simulink model "momentumBasedFlight"  (R2021b)
settings: Solver=FixedStepDiscrete  StartTime=0.0  StopTime=Config.simulationTime  FixedStep=Config.tStep  RelTol=1e-3
InitFcn:
  | cd(fileparts(which(bdroot)));
  | initMomentumBasedFlight;
StopFcn:
  | cd(fileparts(which(bdroot)));
  | stopMomentumBasedFlight;
undefined symbols (not defined in the file or in its folder): Config
libraries: WBToolboxLibrary x18, momentum_flight_control_v1 x6, thrust_estimation_v1 x1, jets_control_v1 x1
settings Model: NumberOfSteps=50  Creator=gnava  LastModifiedBy=gnava
settings SolverCC: AlgebraicLoopSolver=TrustRegion
settings DataIOCC: ReturnWorkspaceOutputs=off
settings OptimizationCC: BlockReduction=off  DefaultParameterBehavior=Inlined  BufferReuse=off
settings DebuggingCC: SFMachineParentedDataDiag=warning  ArithmeticOperatorsInVariantConditions=warning
settings SFSimCC: SimUseLocalCustomCode=off  CustomCodeUndefinedFunction=UseInterfaceOnly
settings RTWCC: RTWUseLocalCustomCode=off

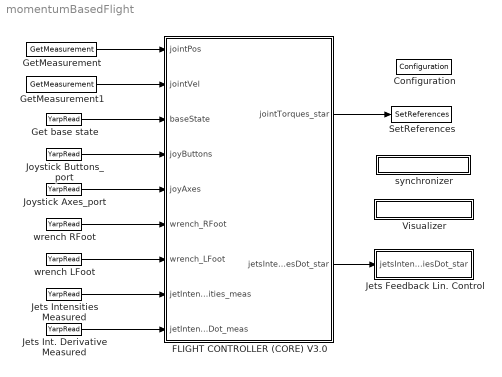
== system momentumBasedFlight ==
  Configuration : WBToolboxLibrary/Utilities/Configuration  ConfigSource=Workspace  ConfigObject='WBTConfigRobot'  RobotName='icubSim'  UrdfFile='model.urdf'  ControlledJoints={'l_elbow','l_shoulder_pitch','torso_roll'}  ControlBoardsNames={'left_arm','right_arm','torso'}  LocalName='WBT'  GravityVector=[0,0,-9.81]
      settings: SourceProductName=WholeBodyToolbox
  FLIGHT CONTROLLER (CORE) V3.0 : Subsystem
  Get base state : WBToolboxLibrary/Utilities/YarpRead  portName=Ports.BASE_STATE  signalSize=18  timeout=0.5  blocking=off  timestamp=off  autoconnect=on  errorOnConnection=on
      settings: SourceProductName=WholeBodyToolbox
  GetMeasurement : WBToolboxLibrary/States/GetMeasurement  measuredType=Joints Position
      settings: SourceProductName=WholeBodyToolbox
  GetMeasurement1 : WBToolboxLibrary/States/GetMeasurement  measuredType=Joints Velocity
      settings: SourceProductName=WholeBodyToolbox
  Jets Feedback Lin. Control : Subsystem
  Jets Int. Derivative Measured : WBToolboxLibrary/Utilities/YarpRead  portName=Ports.THRUST_DOT  signalSize=4  timeout=0.5  blocking=off  timestamp=off  autoconnect=on  errorOnConnection=off
      settings: SourceProductName=WholeBodyToolbox
  Jets Intensities Measured : WBToolboxLibrary/Utilities/YarpRead  portName=Ports.JETS_THRUSTS  signalSize=4  timeout=0.5  blocking=off  timestamp=off  autoconnect=on  errorOnConnection=on
      settings: SourceProductName=WholeBodyToolbox
  Joystick Axes_port : WBToolboxLibrary/Utilities/YarpRead  portName=Ports.JOYSTICK_AXIS  signalSize=6  timeout=0.5  blocking=off  timestamp=off  autoconnect=on  errorOnConnection=off
      settings: SourceProductName=WholeBodyToolbox
  Joystick Buttons_port : WBToolboxLibrary/Utilities/YarpRead  portName=Ports.JOYSTICK_BUTTONS  signalSize=24  timeout=0.5  blocking=off  timestamp=off  autoconnect=on  errorOnConnection=off
      settings: SourceProductName=WholeBodyToolbox
  SetReferences : WBToolboxLibrary/Actuators/SetReferences  controlType=Torque  refSpeed=10*(pi/180)  refAcceleration=1000000*(pi/180)
      settings: SourceProductName=WholeBodyToolbox
  Visualizer : Subsystem
      mask Display: disp('VISUALIZER')
  synchronizer : Subsystem
      mask Display: disp('SYNCHRONIZER')
  wrench LFoot : WBToolboxLibrary/Utilities/YarpRead  portName=Ports.WRENCH_LEFT_FOOT  signalSize=6  timeout=0.5  blocking=off  timestamp=off  autoconnect=on  errorOnConnection=on
      settings: SourceProductName=WholeBodyToolbox
  wrench RFoot : WBToolboxLibrary/Utilities/YarpRead  portName=Ports.WRENCH_RIGHT_FOOT  signalSize=6  timeout=0.5  blocking=off  timestamp=off  autoconnect=on  errorOnConnection=on
      settings: SourceProductName=WholeBodyToolbox
  wires:
  GetMeasurement/1 -> FLIGHT CONTROLLER (CORE) V3.0/1(jointPos)
  GetMeasurement1/1 -> FLIGHT CONTROLLER (CORE) V3.0/2(jointVel)
  Joystick Buttons_port/1 -> FLIGHT CONTROLLER (CORE) V3.0/4(joyButtons)
  Joystick Axes_port/1 -> FLIGHT CONTROLLER (CORE) V3.0/5(joyAxes)
  Get base state/1 -> FLIGHT CONTROLLER (CORE) V3.0/3(baseState)
  wrench LFoot/1 -> FLIGHT CONTROLLER (CORE) V3.0/7(wrench_LFoot)
  wrench RFoot/1 -> FLIGHT CONTROLLER (CORE) V3.0/6(wrench_RFoot)
  FLIGHT CONTROLLER (CORE) V3.0/1(jointTorques_star) -> SetReferences/1
  Jets Int. Derivative Measured/1 -> FLIGHT CONTROLLER (CORE) V3.0/9(jetIntensitiesDot_meas)
  FLIGHT CONTROLLER (CORE) V3.0/2(jetsIntensitiesDot_star) -> Jets Feedback Lin. Control/1(jetsIntensitiesDot_star)
  Jets Intensities Measured/1 -> FLIGHT CONTROLLER (CORE) V3.0/8(jetIntensities_meas)

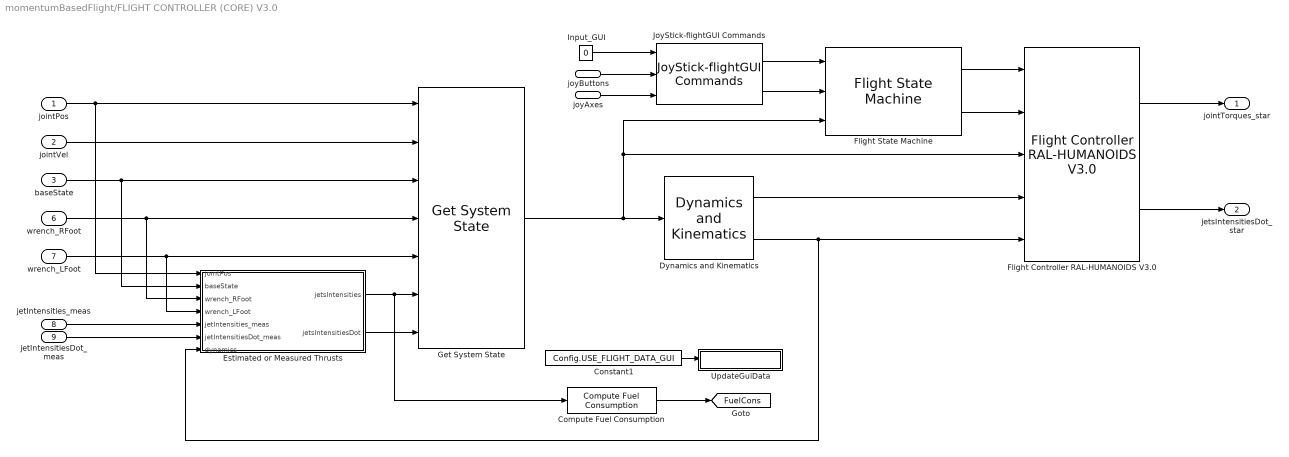
== system momentumBasedFlight/FLIGHT CONTROLLER (CORE) V3.0 ==
  jointPos : Inport
  jointVel : Inport  Port=2
  baseState : Inport  Port=3
  joyButtons : Inport  Port=4
  joyAxes : Inport  Port=5
  wrench_RFoot : Inport  Port=6
  wrench_LFoot : Inport  Port=7
  jetIntensities_meas : Inport  Port=8
  jetIntensitiesDot_meas : Inport  Port=9
  Compute Fuel Consumption : momentum_flight_control_v1/Compute Fuel Consumption  Parameter1=Config
      settings: SourceProductName=iRonCub Library v1
  Constant1 : Constant  Value=Config.USE_FLIGHT_DATA_GUI
  Dynamics and Kinematics : momentum_flight_control_v1/Dynamics and Kinematics  Parameter1=Config  Parameter2=Frames
      settings: SourceProductName=iRonCub Library v1
  Estimated or Measured Thrusts : Subsystem
  Flight Controller RAL-HUMANOIDS V3.0 : momentum_flight_control_v1/Flight Controller RAL-HUMANOIDS V3.0  Parameter1=Config
      settings: SourceProductName=iRonCub Library v1
  Flight State Machine : momentum_flight_control_v1/Flight State Machine  Parameter1=Config  Parameter2=Frames
      settings: SourceProductName=iRonCub Library v1
  Get System State : momentum_flight_control_v1/Get System State  Parameter1=Frames
      settings: SourceProductName=iRonCub Library v1
  Input_GUI : Constant  Value=0
  JoyStick-flightGUI Commands : momentum_flight_control_v1/JoyStick-flightGUI Commands  Parameter1=Config
      settings: SourceProductName=iRonCub Library v1
  UpdateGuiData : Subsystem
      mask Display: disp('Update Data GUI')
  jointTorques_star : Outport  VectorParamsAs1DForOutWhenUnconnected=off
  jetsIntensitiesDot_star : Outport  Port=2  VectorParamsAs1DForOutWhenUnconnected=off
  tag scope: FuelCons=global
  wires:
  wrench_LFoot/1 -> Get System State/5, Estimated or Measured Thrusts/4(wrench_LFoot)
  Flight Controller RAL-HUMANOIDS V3.0/2 -> jetsIntensitiesDot_star/1
  Flight Controller RAL-HUMANOIDS V3.0/1 -> jointTorques_star/1
  Dynamics and Kinematics/1 -> Flight Controller RAL-HUMANOIDS V3.0/4
  Get System State/1 -> Dynamics and Kinematics/1, Flight Controller RAL-HUMANOIDS V3.0/3, Flight State Machine/3
  jointVel/1 -> Get System State/2
  jointPos/1 -> Get System State/1, Estimated or Measured Thrusts/1(jointPos)
  wrench_RFoot/1 -> Get System State/4, Estimated or Measured Thrusts/3(wrench_RFoot)
  baseState/1 -> Get System State/3, Estimated or Measured Thrusts/2(baseState)
  Compute Fuel Consumption/1 -> [FuelCons]
  JoyStick-flightGUI Commands/1 -> Flight State Machine/1
  JoyStick-flightGUI Commands/2 -> Flight State Machine/2
  Flight State Machine/1 -> Flight Controller RAL-HUMANOIDS V3.0/1
  Flight State Machine/2 -> Flight Controller RAL-HUMANOIDS V3.0/2
  joyAxes/1 -> JoyStick-flightGUI Commands/3
  joyButtons/1 -> JoyStick-flightGUI Commands/2
  Input_GUI/1 -> JoyStick-flightGUI Commands/1
  Constant1/1 -> UpdateGuiData/Enable
  Dynamics and Kinematics/2 -> Flight Controller RAL-HUMANOIDS V3.0/5, Estimated or Measured Thrusts/7(dynamics)
  jetIntensities_meas/1 -> Estimated or Measured Thrusts/5(jetIntensities_meas)
  jetIntensitiesDot_meas/1 -> Estimated or Measured Thrusts/6(jetIntensitiesDot_meas)
  Estimated or Measured Thrusts/1(jetsIntensities) -> Compute Fuel Consumption/1, Get System State/6
  Estimated or Measured Thrusts/2(jetsIntensitiesDot) -> Get System State/7

== system momentumBasedFlight/Jets Feedback Lin. Control ==
  jetsIntensitiesDot_star : Inport
  Bus Creator : BusCreator  Inputs=2
  Feedback Linearization Jets Control : jets_control_v1/Feedback linearization 4-jets control  Conf=Config
      settings: SourceProductName=iRonCub Library v1
  Logical Operator : Logic  Operator=NOT  AllPortsSameDT=off  OutDataTypeStr=boolean
  "ON_GAZEBO " : Constant  Value=Config.USE_JET_DYNAMICS
  SET THROTTLE : Subsystem
  SET_THRUST_DERIVATIVE : Subsystem
  tag scope: throttle=global
  wires:
  jetsIntensitiesDot_star/1 -> Feedback Linearization Jets Control/2, SET_THRUST_DERIVATIVE/1(jetsIntensitiesDot_star)
  Feedback Linearization Jets Control/1 -> [throttle], SET THROTTLE/1(throttle)
  Bus Creator/1 -> Feedback Linearization Jets Control/1
  [jetsIntensities] -> Bus Creator/1  "jetIntensitiesFiltered"
  [jetIntensitiesDot] -> Bus Creator/2  "jetDerivativesEst"
  "ON_GAZEBO "/1 -> SET THROTTLE/Enable, Logical Operator/1
  Logical Operator/1 -> SET_THRUST_DERIVATIVE/Enable

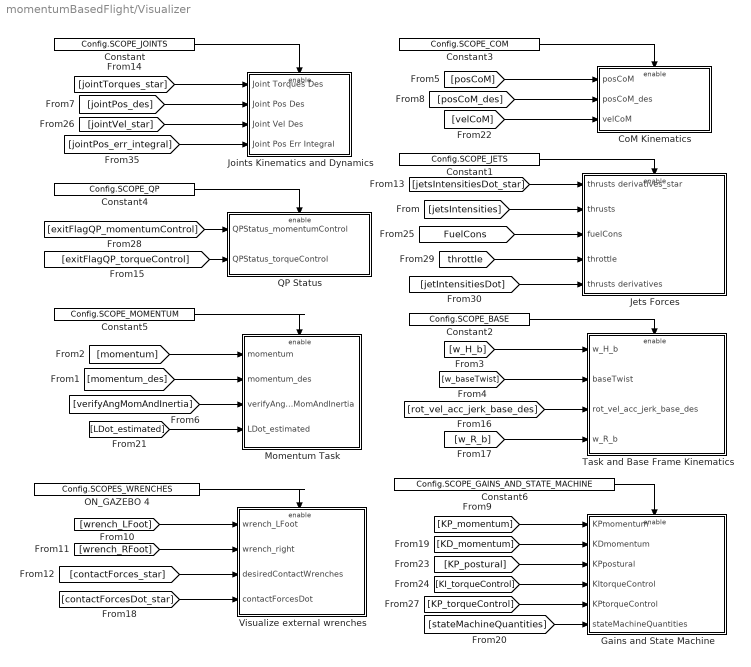
== system momentumBasedFlight/Visualizer ==
  CoM Kinematics : Subsystem
  Constant : Constant  Value=Config.SCOPE_JOINTS
  Constant1 : Constant  Value=Config.SCOPE_JETS
  Constant2 : Constant  Value=Config.SCOPE_BASE
  Constant3 : Constant  Value=Config.SCOPE_COM
  Constant4 : Constant  Value=Config.SCOPE_QP
  Constant5 : Constant  Value=Config.SCOPE_MOMENTUM
  Constant6 : Constant  Value=Config.SCOPE_GAINS_AND_STATE_MACHINE
  Gains and State Machine : Subsystem
  Jets Forces : Subsystem
  Joints Kinematics and Dynamics : Subsystem
  Momentum Task : Subsystem
  ON_GAZEBO 4 : Constant  Value=Config.SCOPES_WRENCHES
  QP Status : Subsystem
  Task and Base Frame Kinematics : Subsystem
  "Visualize external wrenches  " : Subsystem
  wires:
  [jointTorques_star] -> Joints Kinematics and Dynamics/1(Joint Torques Des)
  [jointPos_des] -> Joints Kinematics and Dynamics/2(Joint Pos Des)
  [w_H_b] -> Task and Base Frame Kinematics/1(w_H_b)
  [jointVel_star] -> Joints Kinematics and Dynamics/3(Joint Vel Des)
  Constant/1 -> Joints Kinematics and Dynamics/Enable
  [jetsIntensitiesDot_star] -> Jets Forces/1(thrusts derivatives_star)
  Constant1/1 -> Jets Forces/Enable
  [w_baseTwist] -> Task and Base Frame Kinematics/2(baseTwist)
  Constant2/1 -> Task and Base Frame Kinematics/Enable
  [momentum] -> Momentum Task/1(momentum)
  [posCoM] -> CoM Kinematics/1(posCoM)
  [posCoM_des] -> CoM Kinematics/2(posCoM_des)
  Constant3/1 -> CoM Kinematics/Enable
  [exitFlagQP_momentumControl] -> QP Status/1(QPStatus_momentumControl)
  Constant4/1 -> QP Status/Enable
  Constant5/1 -> Momentum Task/Enable
  [rot_vel_acc_jerk_base_des] -> Task and Base Frame Kinematics/3(rot_vel_acc_jerk_base_des)
  [w_R_b] -> Task and Base Frame Kinematics/4(w_R_b)
  [momentum_des] -> Momentum Task/2(momentum_des)
  [jetsIntensities] -> Jets Forces/2(thrusts)
  [verifyAngMomAndInertia] -> Momentum Task/3(verifyAngMomAndInertia)
  [wrench_LFoot] -> "Visualize external wrenches  "/1(wrench_LFoot)
  [wrench_RFoot] -> "Visualize external wrenches  "/2(wrench_right)
  ON_GAZEBO 4/1 -> "Visualize external wrenches  "/Enable
  [contactForces_star] -> "Visualize external wrenches  "/3(desiredContactWrenches)
  [exitFlagQP_torqueControl] -> QP Status/2(QPStatus_torqueControl)
  [contactForcesDot_star] -> "Visualize external wrenches  "/4(contactForcesDot)
  [LDot_estimated] -> Momentum Task/4(LDot_estimated)
  Constant6/1 -> Gains and State Machine/Enable
  [KP_momentum] -> Gains and State Machine/1(KPmomentum)
  [stateMachineQuantities] -> Gains and State Machine/6(stateMachineQuantities)
  [KD_momentum] -> Gains and State Machine/2(KDmomentum)
  [KP_postural] -> Gains and State Machine/3(KPpostural)
  [KP_torqueControl] -> Gains and State Machine/5(KPtorqueControl)
  [KI_torqueControl] -> Gains and State Machine/4(KItorqueControl)
  [jointPos_err_integral] -> Joints Kinematics and Dynamics/4(Joint Pos Err Integral)
  [velCoM] -> CoM Kinematics/3(velCoM)
  [FuelCons] -> Jets Forces/3(fuelCons)
  [throttle] -> Jets Forces/4(throttle)
  [jetIntensitiesDot] -> Jets Forces/5(thrusts derivatives)

== system momentumBasedFlight/synchronizer ==
  GAZEBO_SYNCHRONIZER : Subsystem
  Logical Operator : Logic  Operator=NOT  AllPortsSameDT=off  OutDataTypeStr=boolean
  "ON_GAZEBO " : Constant  Value=Config.ON_GAZEBO
  REAL_TIME_SYNC : Subsystem
  wires:
  Logical Operator/1 -> REAL_TIME_SYNC/Enable
  "ON_GAZEBO "/1 -> GAZEBO_SYNCHRONIZER/Enable, Logical Operator/1

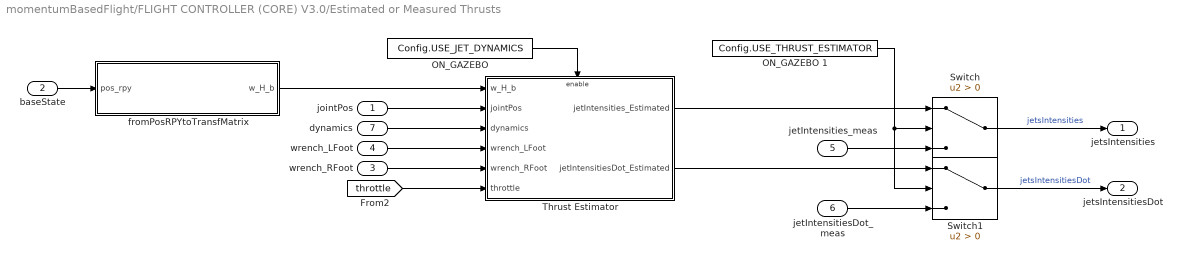
== system momentumBasedFlight/FLIGHT CONTROLLER (CORE) V3.0/Estimated or Measured Thrusts ==
  jointPos : Inport
  baseState : Inport  Port=2
  wrench_RFoot : Inport  Port=3
  wrench_LFoot : Inport  Port=4
  jetIntensities_meas : Inport  Port=5
  jetIntensitiesDot_meas : Inport  Port=6
  dynamics : Inport  Port=7
  " Thrust Estimator" : Subsystem
  "ON_GAZEBO " : Constant  Value=Config.USE_JET_DYNAMICS
  ON_GAZEBO 1 : Constant  Value=Config.USE_THRUST_ESTIMATOR
  Switch : Switch  Criteria=u2 > Threshold
  Switch1 : Switch  Criteria=u2 > Threshold
  fromPosRPYtoTransfMatrix : MATLAB Function  TreatAsAtomicUnit=on
  jetsIntensities : Outport
  jetsIntensitiesDot : Outport  Port=2
  wires:
  Switch/1 -> jetsIntensities/1  "jetsIntensities"
  jetIntensitiesDot_meas/1 -> Switch1/3
  " Thrust Estimator"/1(jetIntensities_Estimated) -> Switch/1
  jetIntensities_meas/1 -> Switch/3
  " Thrust Estimator"/2(jetIntensitiesDot_Estimated) -> Switch1/1
  wrench_RFoot/1 -> " Thrust Estimator"/5(wrench_RFoot)
  ON_GAZEBO 1/1 -> Switch/2, Switch1/2
  jointPos/1 -> " Thrust Estimator"/2(jointPos)
  Switch1/1 -> jetsIntensitiesDot/1  "jetsIntensitiesDot"
  dynamics/1 -> " Thrust Estimator"/3(dynamics)
  [throttle] -> " Thrust Estimator"/6(throttle)
  "ON_GAZEBO "/1 -> " Thrust Estimator"/Enable
  wrench_LFoot/1 -> " Thrust Estimator"/4(wrench_LFoot)
  baseState/1 -> fromPosRPYtoTransfMatrix/1(pos_rpy)
  fromPosRPYtoTransfMatrix/1(w_H_b) -> " Thrust Estimator"/1(w_H_b)

== system momentumBasedFlight/FLIGHT CONTROLLER (CORE) V3.0/UpdateGuiData ==
  Enable : EnablePort
  Clock : Clock
  Update Data for the GUI : MATLAB Function  TreatAsAtomicUnit=on
  wires:
  Clock/1 -> Update Data for the GUI/1(time)

== system momentumBasedFlight/Jets Feedback Lin. Control/SET THROTTLE ==
  throttle : Inport
  Enable : EnablePort
  Set Throttle : WBToolboxLibrary/Utilities/YarpWrite  portName=Ports.THROTTLE  autoconnect=on  errorOnConnection=on
      settings: SourceProductName=WholeBodyToolbox
  wires:
  throttle/1 -> Set Throttle/1

== system momentumBasedFlight/Jets Feedback Lin. Control/SET_THRUST_DERIVATIVE ==
  jetsIntensitiesDot_star : Inport
  Enable : EnablePort
  Set Thrust Derivative : WBToolboxLibrary/Utilities/YarpWrite  portName=Ports.THRUST_RATIO  autoconnect=on  errorOnConnection=on
      settings: SourceProductName=WholeBodyToolbox
  wires:
  jetsIntensitiesDot_star/1 -> Set Thrust Derivative/1

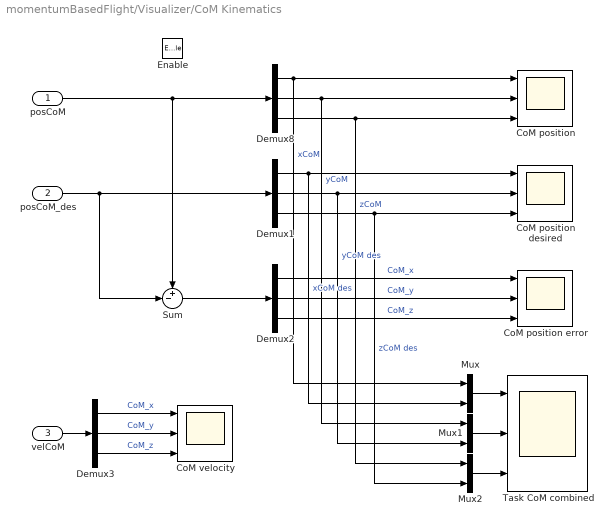
== system momentumBasedFlight/Visualizer/CoM Kinematics ==
  posCoM : Inport
  posCoM_des : Inport  Port=2
  velCoM : Inport  Port=3
  Enable : EnablePort
  CoM position : Scope  NumInputPorts=3
  CoM position desired : Scope  NumInputPorts=3
  CoM position error : Scope  NumInputPorts=3
  CoM velocity : Scope  NumInputPorts=3
  Demux{1..3,8} (4 alike) : Demux  Outputs=3
  Mux : Mux  Inputs=2
  Mux1 : Mux  Inputs=2
  Mux2 : Mux  Inputs=2
  Sum : Sum  Inputs=+-|
  Task CoM combined : Scope  NumInputPorts=3
  wires:
  posCoM/1 -> Sum/1, Demux8/1
  posCoM_des/1 -> Sum/2, Demux1/1
  Sum/1 -> Demux2/1
  Demux2/3 -> CoM position error/3  "CoM_z"
  Demux2/2 -> CoM position error/2  "CoM_y"
  Demux2/1 -> CoM position error/1  "CoM_x"
  Demux8/2 -> CoM position/2, Mux1/1  "yCoM"
  Demux1/2 -> Mux1/2, CoM position desired/2  "yCoM des"
  Mux2/1 -> Task CoM combined/3
  Demux8/1 -> CoM position/1, Mux/1  "xCoM"
  Demux8/3 -> CoM position/3, Mux2/1  "zCoM"
  Mux1/1 -> Task CoM combined/2
  Demux1/1 -> CoM position desired/1, Mux/2  "xCoM des"
  Demux1/3 -> CoM position desired/3, Mux2/2  "zCoM des"
  Mux/1 -> Task CoM combined/1
  velCoM/1 -> Demux3/1
  Demux3/1 -> CoM velocity/1  "CoM_x"
  Demux3/2 -> CoM velocity/2  "CoM_y"
  Demux3/3 -> CoM velocity/3  "CoM_z"

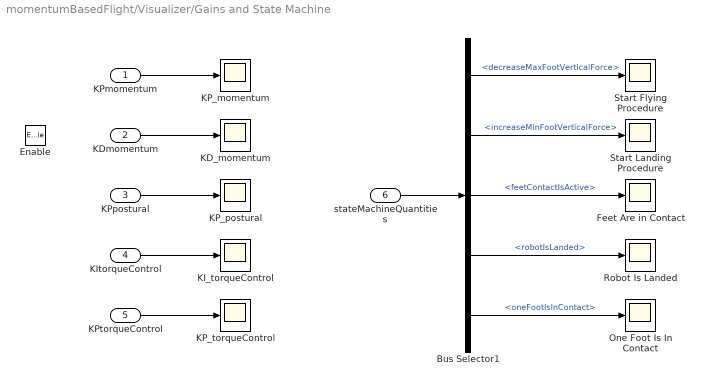
== system momentumBasedFlight/Visualizer/Gains and State Machine ==
  KPmomentum : Inport
  KDmomentum : Inport  Port=2
  KPpostural : Inport  Port=3
  KItorqueControl : Inport  Port=4
  KPtorqueControl : Inport  Port=5
  stateMachineQuantities : Inport  Port=6
  Enable : EnablePort
  Bus Selector1 : BusSelector  OutputSignals=decreaseMaxFootVerticalForce,increaseMinFootVerticalForce,feetContactIsActive,robotIsLanded,oneFootIsInContact
  Feet Are in Contact : Scope
  KD_momentum : Scope
  KI_torqueControl : Scope
  KP_momentum : Scope
  KP_postural : Scope
  KP_torqueControl : Scope
  One Foot Is In Contact : Scope
  Robot Is Landed : Scope
  Start Flying Procedure : Scope
  Start Landing Procedure : Scope
  wires:
  stateMachineQuantities/1 -> Bus Selector1/1
  Bus Selector1/1 -> Start Flying Procedure/1  "<decreaseMaxFootVerticalForce>"
  Bus Selector1/2 -> Start Landing Procedure/1  "<increaseMinFootVerticalForce>"
  Bus Selector1/3 -> Feet Are in Contact/1  "<feetContactIsActive>"
  KPmomentum/1 -> KP_momentum/1
  KDmomentum/1 -> KD_momentum/1
  KPpostural/1 -> KP_postural/1
  KItorqueControl/1 -> KI_torqueControl/1
  KPtorqueControl/1 -> KP_torqueControl/1
  Bus Selector1/4 -> Robot Is Landed/1  "<robotIsLanded>"
  Bus Selector1/5 -> One Foot Is In Contact/1  "<oneFootIsInContact>"

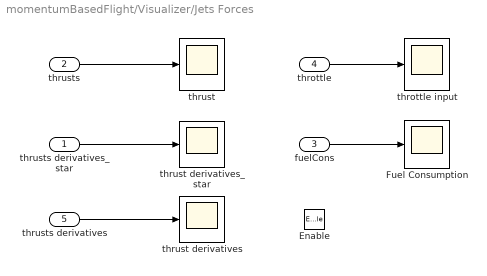
== system momentumBasedFlight/Visualizer/Jets Forces ==
  thrusts derivatives_star : Inport
  thrusts : Inport  Port=2
  fuelCons : Inport  Port=3
  throttle : Inport  Port=4
  thrusts derivatives : Inport  Port=5
  Enable : EnablePort
  Fuel Consumption : Scope
  throttle input : Scope
  thrust : Scope
  thrust derivatives : Scope
  thrust derivatives_star : Scope
  wires:
  thrusts derivatives_star/1 -> thrust derivatives_star/1
  thrusts/1 -> thrust/1
  fuelCons/1 -> Fuel Consumption/1
  throttle/1 -> throttle input/1
  thrusts derivatives/1 -> thrust derivatives/1

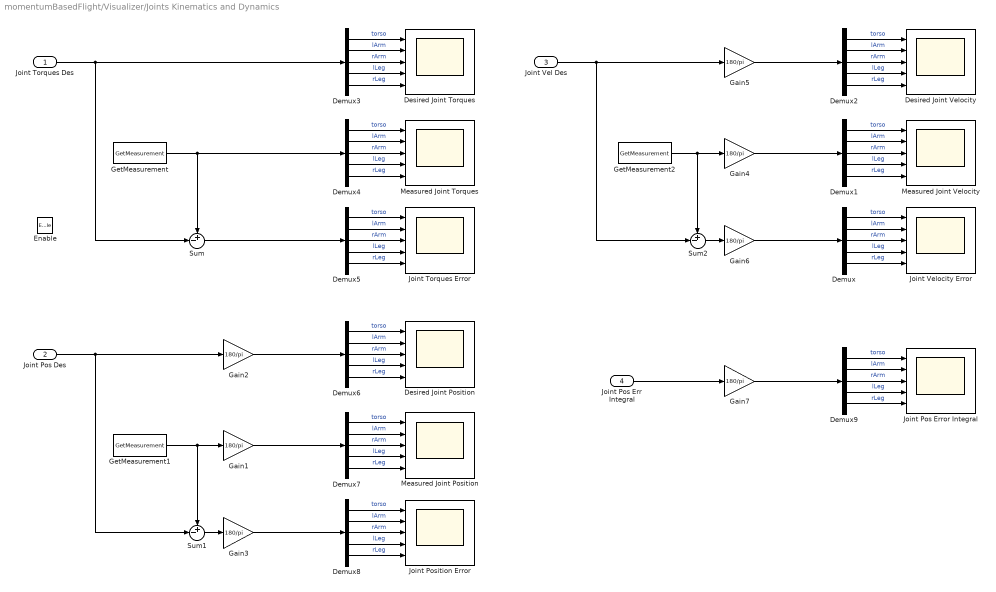
== system momentumBasedFlight/Visualizer/Joints Kinematics and Dynamics ==
  Joint Torques Des : Inport
  Joint Pos Des : Inport  Port=2
  Joint Vel Des : Inport  Port=3
  Joint Pos Err Integral : Inport  Port=4
  Enable : EnablePort
  Demux{,1..9} (10 alike) : Demux  Outputs=Config.numOfJointsForEachControlboard
  Desired Joint Position : Scope  NumInputPorts=5
  Desired Joint Torques : Scope  NumInputPorts=5
  Desired Joint Velocity : Scope  NumInputPorts=5
  Gain{1..7} (7 alike) : Gain  Gain=180/pi
  GetMeasurement : WBToolboxLibrary/States/GetMeasurement  measuredType=Joints Torque
      settings: SourceProductName=WholeBodyToolbox
  GetMeasurement1 : WBToolboxLibrary/States/GetMeasurement  measuredType=Joints Position
      settings: SourceProductName=WholeBodyToolbox
  GetMeasurement2 : WBToolboxLibrary/States/GetMeasurement  measuredType=Joints Velocity
      settings: SourceProductName=WholeBodyToolbox
  Joint Pos Error Integral : Scope  NumInputPorts=5
  Joint Position Error : Scope  NumInputPorts=5
  Joint Torques Error : Scope  NumInputPorts=5
  Joint Velocity Error : Scope  NumInputPorts=5
  Measured Joint Position : Scope  NumInputPorts=5
  Measured Joint Torques : Scope  NumInputPorts=5
  Measured Joint Velocity : Scope  NumInputPorts=5
  Sum : Sum  Inputs=+-|
  Sum1 : Sum  Inputs=+-|
  Sum2 : Sum  Inputs=+-|
  wires:
  Demux5/3 -> Joint Torques Error/3  "rArm"
  Demux5/4 -> Joint Torques Error/4  "lLeg"
  Demux5/5 -> Joint Torques Error/5  "rLeg"
  Sum/1 -> Demux5/1
  Demux5/1 -> Joint Torques Error/1  "torso"
  Demux5/2 -> Joint Torques Error/2  "lArm"
  GetMeasurement/1 -> Demux4/1, Sum/1
  Demux4/3 -> Measured Joint Torques/3  "rArm"
  Demux4/2 -> Measured Joint Torques/2  "lArm"
  Demux4/5 -> Measured Joint Torques/5  "rLeg"
  Demux4/4 -> Measured Joint Torques/4  "lLeg"
  Demux4/1 -> Measured Joint Torques/1  "torso"
  Demux3/1 -> Desired Joint Torques/1  "torso"
  Demux3/5 -> Desired Joint Torques/5  "rLeg"
  Joint Torques Des/1 -> Demux3/1, Sum/2
  Demux3/3 -> Desired Joint Torques/3  "rArm"
  Demux3/2 -> Desired Joint Torques/2  "lArm"
  Demux3/4 -> Desired Joint Torques/4  "lLeg"
  Demux7/4 -> Measured Joint Position/4  "lLeg"
  Demux7/2 -> Measured Joint Position/2  "lArm"
  Joint Pos Des/1 -> Sum1/2, Gain2/1
  Demux8/2 -> Joint Position Error/2  "lArm"
  Sum1/1 -> Gain3/1
  Demux7/1 -> Measured Joint Position/1  "torso"
  Demux8/5 -> Joint Position Error/5  "rLeg"
  GetMeasurement1/1 -> Sum1/1, Gain1/1
  Demux8/4 -> Joint Position Error/4  "lLeg"
  Demux6/1 -> Desired Joint Position/1  "torso"
  Demux8/3 -> Joint Position Error/3  "rArm"
  Demux6/2 -> Desired Joint Position/2  "lArm"
  Demux6/4 -> Desired Joint Position/4  "lLeg"
  Demux7/5 -> Measured Joint Position/5  "rLeg"
  Demux6/5 -> Desired Joint Position/5  "rLeg"
  Demux8/1 -> Joint Position Error/1  "torso"
  Demux7/3 -> Measured Joint Position/3  "rArm"
  Demux6/3 -> Desired Joint Position/3  "rArm"
  Gain1/1 -> Demux7/1
  Gain2/1 -> Demux6/1
  Gain3/1 -> Demux8/1
  Joint Vel Des/1 -> Sum2/2, Gain5/1
  Demux2/3 -> Desired Joint Velocity/3  "rArm"
  Demux/3 -> Joint Velocity Error/3  "rArm"
  Demux2/1 -> Desired Joint Velocity/1  "torso"
  Demux2/5 -> Desired Joint Velocity/5  "rLeg"
  Demux2/4 -> Desired Joint Velocity/4  "lLeg"
  Demux1/5 -> Measured Joint Velocity/5  "rLeg"
  Demux1/1 -> Measured Joint Velocity/1  "torso"
  Demux/5 -> Joint Velocity Error/5  "rLeg"
  Gain4/1 -> Demux1/1
  Demux/2 -> Joint Velocity Error/2  "lArm"
  Demux/1 -> Joint Velocity Error/1  "torso"
  Demux/4 -> Joint Velocity Error/4  "lLeg"
  Sum2/1 -> Gain6/1
  Demux1/2 -> Measured Joint Velocity/2  "lArm"
  Demux1/4 -> Measured Joint Velocity/4  "lLeg"
  Demux2/2 -> Desired Joint Velocity/2  "lArm"
  Demux1/3 -> Measured Joint Velocity/3  "rArm"
  Gain6/1 -> Demux/1
  Gain5/1 -> Demux2/1
  GetMeasurement2/1 -> Sum2/1, Gain4/1
  Demux9/1 -> Joint Pos Error Integral/1  "torso"
  Demux9/5 -> Joint Pos Error Integral/5  "rLeg"
  Joint Pos Err Integral/1 -> Gain7/1
  Gain7/1 -> Demux9/1
  Demux9/3 -> Joint Pos Error Integral/3  "rArm"
  Demux9/2 -> Joint Pos Error Integral/2  "lArm"
  Demux9/4 -> Joint Pos Error Integral/4  "lLeg"

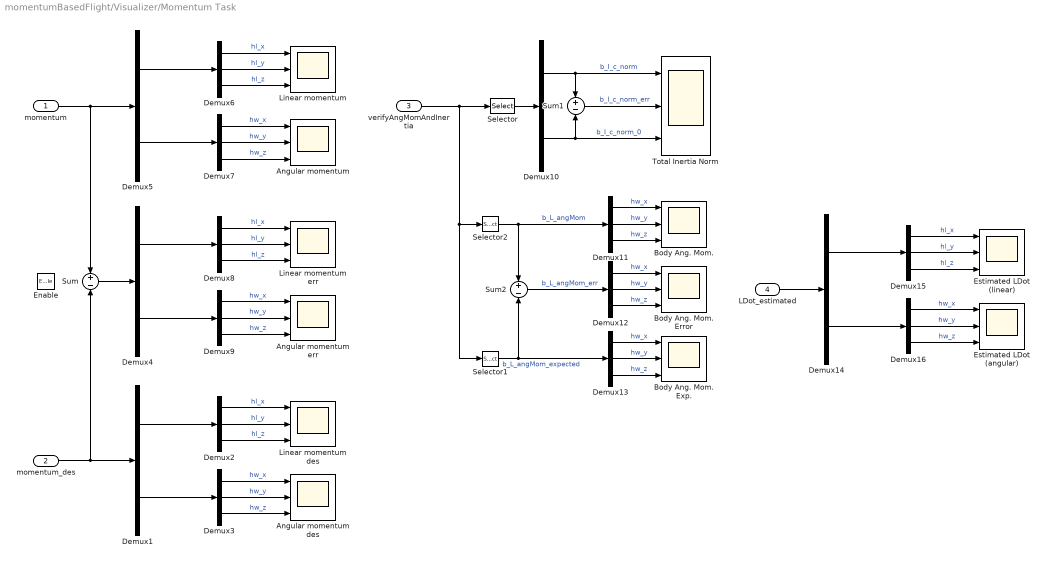
== system momentumBasedFlight/Visualizer/Momentum Task ==
  momentum : Inport
  momentum_des : Inport  Port=2
  verifyAngMomAndInertia : Inport  Port=3
  LDot_estimated : Inport  Port=4
  Enable : EnablePort
  Angular momentum : Scope  NumInputPorts=3
  Angular momentum des : Scope  NumInputPorts=3
  Angular momentum err : Scope  NumInputPorts=3
  Body Ang. Mom. : Scope  NumInputPorts=3
  Body Ang. Mom. Error : Scope  NumInputPorts=3
  Body Ang. Mom. Exp. : Scope  NumInputPorts=3
  Demux{1,4..5,10,14} (5 alike) : Demux  Outputs=2
  Demux{2..3,6..9,11..13,15..16} (11 alike) : Demux  Outputs=3
  Estimated LDot (angular) : Scope  NumInputPorts=3
  Estimated LDot (linear) : Scope  NumInputPorts=3
  Linear momentum : Scope  NumInputPorts=3
  Linear momentum des : Scope  NumInputPorts=3
  Linear momentum err : Scope  NumInputPorts=3
  Selector : Selector  NumberOfDimensions=2  InputPortWidth=3  IndexOptions=Index vector (dialog),Index vector (dialog)  Indices=[1],[1 2]  OutputSizes=1,1
  Selector1 : Selector  NumberOfDimensions=2  InputPortWidth=3  IndexOptions=Index vector (dialog),Index vector (dialog)  Indices=[2 3 4],[2]  OutputSizes=1,1
  Selector2 : Selector  NumberOfDimensions=2  InputPortWidth=3  IndexOptions=Index vector (dialog),Index vector (dialog)  Indices=[2 3 4],[1]  OutputSizes=1,1
  Sum : Sum  Inputs=+|-
  Sum1 : Sum  Inputs=+|-
  Sum2 : Sum  Inputs=+|-
  Total Inertia Norm : Scope  NumInputPorts=3
  wires:
  Demux6/1 -> Linear momentum/1  "hl_x"
  Demux6/3 -> Linear momentum/3  "hl_z"
  Demux5/2 -> Demux7/1
  Demux6/2 -> Linear momentum/2  "hl_y"
  Demux5/1 -> Demux6/1
  Demux7/1 -> Angular momentum/1  "hw_x"
  Demux7/3 -> Angular momentum/3  "hw_z"
  Demux7/2 -> Angular momentum/2  "hw_y"
  momentum/1 -> Sum/1, Demux5/1
  Demux3/2 -> Angular momentum des/2  "hw_y"
  Demux3/1 -> Angular momentum des/1  "hw_x"
  Demux2/3 -> Linear momentum des/3  "hl_z"
  Demux2/1 -> Linear momentum des/1  "hl_x"
  Demux1/2 -> Demux3/1
  Demux1/1 -> Demux2/1
  Demux3/3 -> Angular momentum des/3  "hw_z"
  Demux2/2 -> Linear momentum des/2  "hl_y"
  momentum_des/1 -> Sum/2, Demux1/1
  Demux9/2 -> Angular momentum err/2  "hw_y"
  Demux9/1 -> Angular momentum err/1  "hw_x"
  Demux8/3 -> Linear momentum err/3  "hl_z"
  Demux8/1 -> Linear momentum err/1  "hl_x"
  Demux4/2 -> Demux9/1
  Demux4/1 -> Demux8/1
  Demux9/3 -> Angular momentum err/3  "hw_z"
  Demux8/2 -> Linear momentum err/2  "hl_y"
  Sum/1 -> Demux4/1
  verifyAngMomAndInertia/1 -> Selector/1, Selector1/1, Selector2/1
  Selector/1 -> Demux10/1
  Demux10/1 -> Total Inertia Norm/1, Sum1/1  "b_I_c_norm"
  Demux10/2 -> Total Inertia Norm/3, Sum1/2  "b_I_c_norm_0"
  Sum1/1 -> Total Inertia Norm/2  "b_I_c_norm_err"
  Selector2/1 -> Demux11/1, Sum2/1  "b_L_angMom"
  Demux11/2 -> Body Ang. Mom./2  "hw_y"
  Demux11/3 -> Body Ang. Mom./3  "hw_z"
  Demux11/1 -> Body Ang. Mom./1  "hw_x"
  Demux12/2 -> Body Ang. Mom. Error/2  "hw_y"
  Sum2/1 -> Demux12/1  "b_L_angMom_err"
  Demux12/3 -> Body Ang. Mom. Error/3  "hw_z"
  Demux12/1 -> Body Ang. Mom. Error/1  "hw_x"
  Demux13/2 -> Body Ang. Mom. Exp./2  "hw_y"
  Selector1/1 -> Sum2/2, Demux13/1  "b_L_angMom_expected"
  Demux13/3 -> Body Ang. Mom. Exp./3  "hw_z"
  Demux13/1 -> Body Ang. Mom. Exp./1  "hw_x"
  LDot_estimated/1 -> Demux14/1
  Demux15/3 -> Estimated LDot (linear)/3  "hl_z"
  Demux16/2 -> Estimated LDot (angular)/2  "hw_y"
  Demux14/1 -> Demux15/1
  Demux14/2 -> Demux16/1
  Demux15/2 -> Estimated LDot (linear)/2  "hl_y"
  Demux15/1 -> Estimated LDot (linear)/1  "hl_x"
  Demux16/1 -> Estimated LDot (angular)/1  "hw_x"
  Demux16/3 -> Estimated LDot (angular)/3  "hw_z"

== system momentumBasedFlight/Visualizer/QP Status ==
  QPStatus_momentumControl : Inport
  QPStatus_torqueControl : Inport  Port=2
  Enable : EnablePort
  QP momentum : Scope
  QP torques : Scope
  wires:
  QPStatus_momentumControl/1 -> QP momentum/1
  QPStatus_torqueControl/1 -> QP torques/1

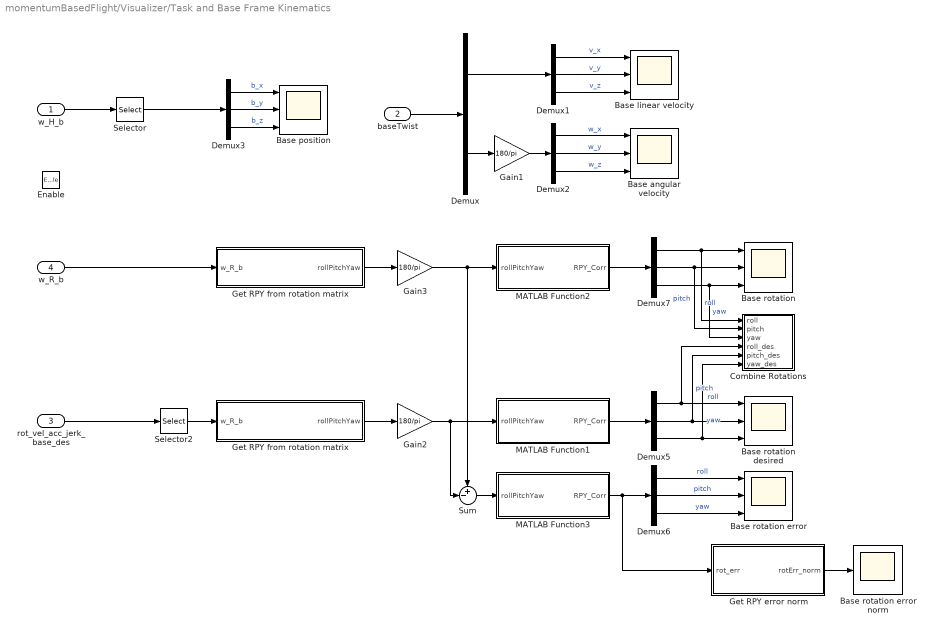
== system momentumBasedFlight/Visualizer/Task and Base Frame Kinematics ==
  w_H_b : Inport
  baseTwist : Inport  Port=2
  rot_vel_acc_jerk_base_des : Inport  Port=3
  w_R_b : Inport  Port=4
  Enable : EnablePort
  Base angular velocity : Scope  NumInputPorts=3
  Base linear velocity : Scope  NumInputPorts=3
  Base position : Scope  NumInputPorts=3
  Base rotation : Scope  NumInputPorts=3
  Base rotation desired : Scope  NumInputPorts=3
  Base rotation error : Scope  NumInputPorts=3
  Base rotation error norm : Scope
  Combine Rotations : Subsystem
  Demux : Demux  Outputs=2
  Demux{1..3,5..7} (6 alike) : Demux  Outputs=3
  Gain1 : Gain  Gain=180/pi
  Gain2 : Gain  Gain=180/pi
  Gain3 : Gain  Gain=180/pi
  Get RPY error norm : MATLAB Function  TreatAsAtomicUnit=on
  Get RPY from rotation matrix : MATLAB Function  TreatAsAtomicUnit=on
  "Get RPY from rotation matrix " : MATLAB Function  TreatAsAtomicUnit=on
  MATLAB Function1 : MATLAB Function  TreatAsAtomicUnit=on
  MATLAB Function2 : MATLAB Function  TreatAsAtomicUnit=on
  MATLAB Function3 : MATLAB Function  TreatAsAtomicUnit=on
  Selector : Selector  NumberOfDimensions=2  InputPortWidth=3  IndexOptions=Index vector (dialog),Index vector (dialog)  Indices=[1:3],4  OutputSizes=1,1
  Selector2 : Selector  NumberOfDimensions=2  InputPortWidth=3  IndexOptions=Index vector (dialog),Index vector (dialog)  Indices=[1:3],[1:3]  OutputSizes=1,1
  Sum : Sum  Inputs=+-|
  wires:
  Demux3/1 -> Base position/1  "b_x"
  Demux3/3 -> Base position/3  "b_z"
  Demux3/2 -> Base position/2  "b_y"
  Selector/1 -> Demux3/1
  w_H_b/1 -> Selector/1
  Demux1/1 -> Base linear velocity/1  "v_x"
  Demux1/3 -> Base linear velocity/3  "v_z"
  Demux2/3 -> Base angular velocity/3  "w_z"
  Demux/2 -> Gain1/1
  Demux2/1 -> Base angular velocity/1  "w_x"
  Demux/1 -> Demux1/1
  Demux2/2 -> Base angular velocity/2  "w_y"
  Gain1/1 -> Demux2/1
  Demux1/2 -> Base linear velocity/2  "v_y"
  "Get RPY from rotation matrix "/1(rollPitchYaw) -> Gain2/1
  Demux5/1 -> Combine Rotations/4(roll_des), Base rotation desired/1  "roll"
  Gain2/1 -> MATLAB Function1/1(rollPitchYaw), Sum/2
  Demux5/2 -> Combine Rotations/5(pitch_des), Base rotation desired/2  "pitch"
  Selector2/1 -> "Get RPY from rotation matrix "/1(w_R_b)
  Demux5/3 -> Combine Rotations/6(yaw_des), Base rotation desired/3  "yaw"
  Demux6/2 -> Base rotation error/2  "pitch"
  Demux6/1 -> Base rotation error/1  "roll"
  Demux6/3 -> Base rotation error/3  "yaw"
  Sum/1 -> MATLAB Function3/1(rollPitchYaw)
  baseTwist/1 -> Demux/1
  rot_vel_acc_jerk_base_des/1 -> Selector2/1
  Gain3/1 -> MATLAB Function2/1(rollPitchYaw), Sum/1
  Demux7/2 -> Combine Rotations/2(pitch), Base rotation/2  "pitch"
  Get RPY from rotation matrix/1(rollPitchYaw) -> Gain3/1
  Demux7/1 -> Combine Rotations/1(roll), Base rotation/1  "roll"
  Demux7/3 -> Combine Rotations/3(yaw), Base rotation/3  "yaw"
  w_R_b/1 -> Get RPY from rotation matrix/1(w_R_b)
  Get RPY error norm/1(rotErr_norm) -> Base rotation error norm/1
  MATLAB Function3/1(RPY_Corr) -> Demux6/1, Get RPY error norm/1(rot_err)
  MATLAB Function1/1(RPY_Corr) -> Demux5/1
  MATLAB Function2/1(RPY_Corr) -> Demux7/1

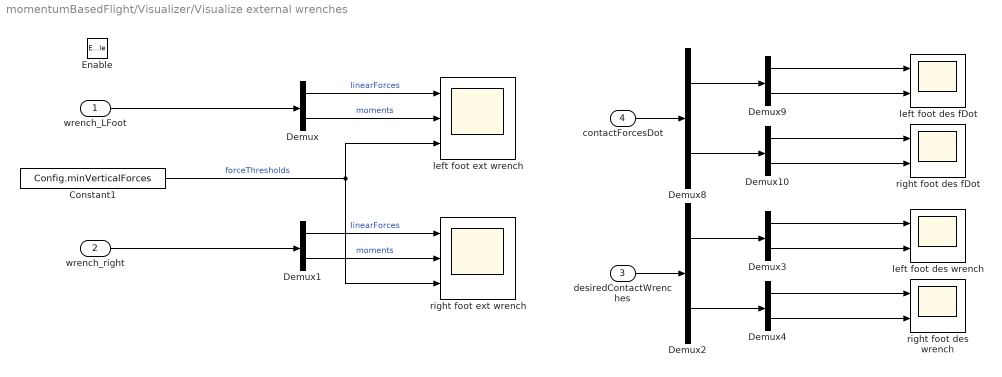
== system momentumBasedFlight/Visualizer/Visualize external wrenches   ==
  wrench_LFoot : Inport
  wrench_right : Inport  Port=2
  desiredContactWrenches : Inport  Port=3
  contactForcesDot : Inport  Port=4
  Enable : EnablePort
  Constant1 : Constant  Value=Config.minVerticalForces
  Demux{,1,3..4,9..10} (6 alike) : Demux  Outputs=[3;3]
  Demux2 : Demux  Outputs=[6;6]
  Demux8 : Demux  Outputs=[6;6]
  left foot des fDot : Scope  NumInputPorts=2
  left foot des wrench : Scope  NumInputPorts=2
  left foot ext wrench : Scope  NumInputPorts=3
  right foot des fDot : Scope  NumInputPorts=2
  right foot des wrench : Scope  NumInputPorts=2
  right foot ext wrench : Scope  NumInputPorts=3
  wires:
  Demux/1 -> left foot ext wrench/1  "linearForces"
  Demux/2 -> left foot ext wrench/2  "moments"
  Demux1/1 -> right foot ext wrench/1  "linearForces"
  Demux1/2 -> right foot ext wrench/2  "moments"
  wrench_LFoot/1 -> Demux/1
  wrench_right/1 -> Demux1/1
  desiredContactWrenches/1 -> Demux2/1
  Demux2/1 -> Demux3/1
  Demux2/2 -> Demux4/1
  Demux4/1 -> right foot des wrench/1
  Demux4/2 -> right foot des wrench/2
  Demux3/1 -> left foot des wrench/1
  Demux3/2 -> left foot des wrench/2
  Demux8/2 -> Demux10/1
  contactForcesDot/1 -> Demux8/1
  Demux10/2 -> right foot des fDot/2
  Demux8/1 -> Demux9/1
  Demux10/1 -> right foot des fDot/1
  Demux9/2 -> left foot des fDot/2
  Demux9/1 -> left foot des fDot/1
  Constant1/1 -> right foot ext wrench/3, left foot ext wrench/3  "forceThresholds"

== system momentumBasedFlight/synchronizer/GAZEBO_SYNCHRONIZER ==
  Enable : EnablePort
  Simulator Synchronizer : WBToolboxLibrary/Utilities/Simulator Synchronizer  period=Config.tStep  serverPortName='/clock/rpc'  clientPortName='/WBT_synchronizer/rpc:o'
      settings: SourceProductName=WholeBodyToolbox

== system momentumBasedFlight/synchronizer/REAL_TIME_SYNC ==
  Enable : EnablePort
  Real Time Synchronizer : WBToolboxLibrary/Utilities/Real Time Synchronizer  period=Config.tStep
      settings: SourceProductName=WholeBodyToolbox

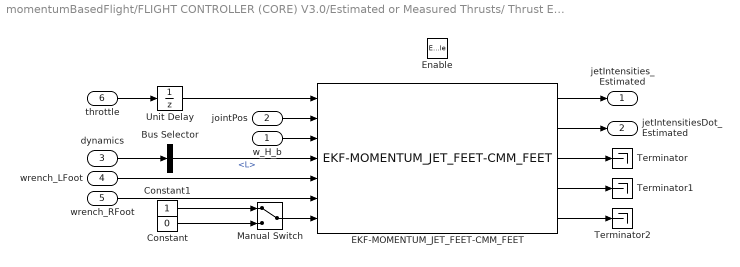
== system momentumBasedFlight/FLIGHT CONTROLLER (CORE) V3.0/Estimated or Measured Thrusts/ Thrust Estimator ==
  w_H_b : Inport
  jointPos : Inport  Port=2
  dynamics : Inport  Port=3
  wrench_LFoot : Inport  Port=4
  wrench_RFoot : Inport  Port=5
  throttle : Inport  Port=6
  Enable : EnablePort
  Bus Selector : BusSelector  OutputSignals=L
  Constant : Constant  Value=0
  Constant1 : Constant
  EKF-MOMENTUM_JET_FEET-CMM_FEET : thrust_estimation_v1/EKF-MOMENTUM_JET_FEET-CMM_FEET  Ts=Config.tStep  Frames=Frames  T0=[0.0; 0.0; 0.0; 0.0]  dot_T0=[0.0; 0.0; 0.0; 0.0]  h0=[0.0; 0.0; 0.0; 0.0; 0.0; 0.0]  fLF0=[0.0; 0.0; 0.0; 0.0; 0.0; 0.0]  fRF0=[0.0; 0.0; 0.0; 0.0; 0.0; 0.0]  P0=blkdiag(eye(4)*1e1, eye(4)*1e1, eye(6)*1e1, eye(6)*1e1, eye(6)*1e1)  Q=blkdiag(eye(4)*1e1, eye(4)*1e1, eye(6)*1e1, eye(6)*1e1, eye(6)*1e1)  R=blkdiag(eye(6)*1e1, eye(6)*1e1, eye(6)*1e1)  jetC_P100=Config.jetC_P100  jetC_P220=Config.jetC_P220
      settings: SourceProductName=iRonCub Library v1
  Manual Switch : ManualSwitch
  Terminator : Terminator
  Terminator1 : Terminator
  Terminator2 : Terminator
  Unit Delay : UnitDelay  SampleTime=-1  HasFrameUpgradeWarning=on
  jetIntensities_Estimated : Outport
  jetIntensitiesDot_Estimated : Outport  Port=2
  wires:
  Unit Delay/1 -> EKF-MOMENTUM_JET_FEET-CMM_FEET/1
  wrench_RFoot/1 -> EKF-MOMENTUM_JET_FEET-CMM_FEET/6
  wrench_LFoot/1 -> EKF-MOMENTUM_JET_FEET-CMM_FEET/5
  EKF-MOMENTUM_JET_FEET-CMM_FEET/5 -> Terminator2/1
  EKF-MOMENTUM_JET_FEET-CMM_FEET/4 -> Terminator1/1
  EKF-MOMENTUM_JET_FEET-CMM_FEET/3 -> Terminator/1
  jointPos/1 -> EKF-MOMENTUM_JET_FEET-CMM_FEET/2
  w_H_b/1 -> EKF-MOMENTUM_JET_FEET-CMM_FEET/3
  throttle/1 -> Unit Delay/1
  EKF-MOMENTUM_JET_FEET-CMM_FEET/2 -> jetIntensitiesDot_Estimated/1
  EKF-MOMENTUM_JET_FEET-CMM_FEET/1 -> jetIntensities_Estimated/1
  Bus Selector/1 -> EKF-MOMENTUM_JET_FEET-CMM_FEET/4  "<L>"
  dynamics/1 -> Bus Selector/1
  Manual Switch/1 -> EKF-MOMENTUM_JET_FEET-CMM_FEET/7
  Constant/1 -> Manual Switch/2
  Constant1/1 -> Manual Switch/1

== system momentumBasedFlight/Visualizer/Task and Base Frame Kinematics/Combine Rotations ==
  roll : Inport
  pitch : Inport  Port=2
  yaw : Inport  Port=3
  roll_des : Inport  Port=4
  pitch_des : Inport  Port=5
  yaw_des : Inport  Port=6
  Mux : Mux  Inputs=2
  Mux1 : Mux  Inputs=2
  Mux2 : Mux  Inputs=2
  Task rotation combined : Scope  NumInputPorts=3
  wires:
  yaw_des/1 -> Mux2/2
  pitch_des/1 -> Mux1/2
  pitch/1 -> Mux1/1
  roll/1 -> Mux/1
  yaw/1 -> Mux2/1
  roll_des/1 -> Mux/2
  Mux2/1 -> Task rotation combined/3
  Mux1/1 -> Task rotation combined/2
  Mux/1 -> Task rotation combined/1

== matlab function momentumBasedFlight/Visualizer/Task and Base Frame Kinematics/MATLAB Function3 ==
  data: RPY_Corr output; rollPitchYaw input
function RPY_Corr = correctYawAngleFCN(rollPitchYaw)

    RPY_Corr = correctYawAngle(rollPitchYaw);

end

== matlab function momentumBasedFlight/Visualizer/Task and Base Frame Kinematics/Get RPY from rotation matrix  ==
  data: w_R_b input; rollPitchYaw output
function rollPitchYaw = rollPitchYawFromRotationFCN(w_R_b)

rollPitchYaw = wbc.rollPitchYawFromRotation(w_R_b);

end

== matlab function momentumBasedFlight/FLIGHT CONTROLLER (CORE) V3.0/Estimated or Measured Thrusts/fromPosRPYtoTransfMatrix ==
  data: pos_rpy input; w_H_b output
function w_H_b = fromPosRpyToTransfMatrixFCN(pos_rpy)

    w_H_b = wbc.fromPosRpyToTransfMatrix(pos_rpy);
end

== matlab function momentumBasedFlight/Visualizer/Task and Base Frame Kinematics/Get RPY from rotation matrix ==
  data: w_R_b input; rollPitchYaw output
function rollPitchYaw = rollPitchYawFromRotationFCN(w_R_b)

rollPitchYaw = wbc.rollPitchYawFromRotation(w_R_b);

end

== matlab function momentumBasedFlight/Visualizer/Task and Base Frame Kinematics/Get RPY error norm ==
  data: rot_err input; rotErr_norm output
function rotErr_norm = normFCN(rot_err)

rotErr_norm = norm(rot_err);

end

== matlab function momentumBasedFlight/Visualizer/Task and Base Frame Kinematics/MATLAB Function2 ==
  data: RPY_Corr output; rollPitchYaw input
function RPY_Corr = correctYawAngleFCN(rollPitchYaw)

    RPY_Corr = correctYawAngle(rollPitchYaw);

end

== matlab function momentumBasedFlight/FLIGHT CONTROLLER (CORE) V3.0/UpdateGuiData/Update Data for the GUI ==
  data: time input
function updateVisualGuiFCN(time)

    coder.extrinsic('updateVisualGui')

    persistent updateTime

    % for now I hard-coded 0.25 [s] as updating time for the data GUI
    timeStepGui    = 0.25;

    if isempty(updateTime)
    
        updateTime = timeStepGui;
    end
    
    % update data GUI
    if time > updateTime
    
        updateVisualGui;
        updateTime = time + timeStepGui;  
    end
end

== matlab function momentumBasedFlight/Visualizer/Task and Base Frame Kinematics/MATLAB Function1 ==
  data: RPY_Corr output; rollPitchYaw input
function RPY_Corr = correctYawAngleFCN(rollPitchYaw)

    RPY_Corr = correctYawAngle(rollPitchYaw);

end
